simulink model "ex3_k_ss_regulator_sim"  (R2023b)
settings: Solver=ode45  StartTime=0.0  StopTime=t_fin  MaxStep=0.01  RelTol=1e-3
values from neighbouring files (symbols this model uses):
  k = [-20.4 -145.89 -335.994]    [basic_variables.mat]    (also in ex3.m = acker(A, B, sb_vec(i)*ones(1, 3)); ex5.m = acker(A, B, [sb sb sb]); ex6.m = acker(A, B, [sb sb sb]); ex7.m = acker(A, B, [sb sb sb]))
  x_0 = [5 -1 3]    [ex3.m]    (also in ex5.m; ex6.m; ex7.m; extra_ex.m)
settings Model: Creator=vistek528  LastModifiedBy=vistek528
settings DataIOCC: ReturnWorkspaceOutputs=off

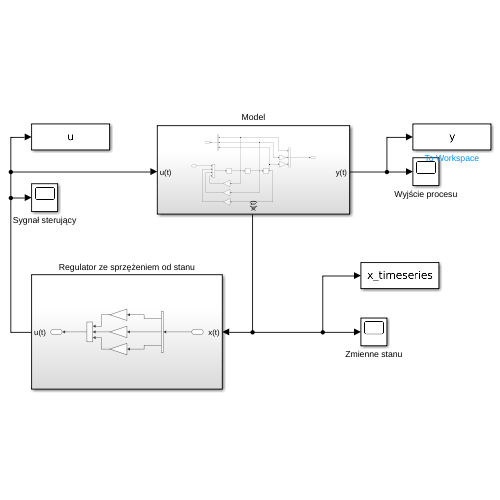
[thumbnail: Simulink's stored preview of the top-level diagram]
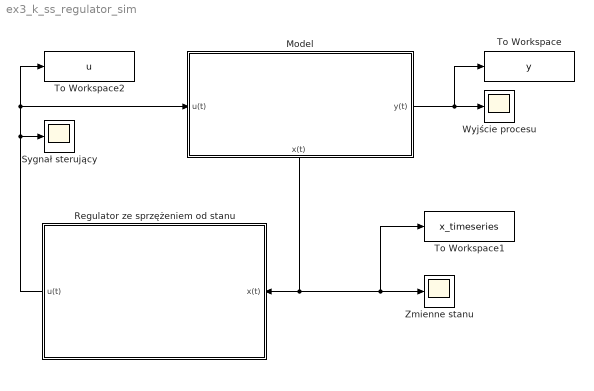
== system ex3_k_ss_regulator_sim ==
  Model : Subsystem
      settings: PortSchema="{\"entries\":[{\"content\":{\"sides\":[{\"content\":{\"connectorIds\":[\"In1\"]},\"type\":\"ConnectorPlacement.EquallySpacedRectSide\",\"uuid\":\"005622f6-1dbe-4fa8-b059-9458e8899b96\"},{\"content\":{\"connectorIds\":[\"Out1\"],\"side\":\"RIGHT\"},\"type\":\"ConnectorPlacement.EquallySpacedRectSide\",\"uuid\":\"7350b0ed-336f-40bc-b296-6ad5a9a87142\"},{\"content\":{\"side\":\"TOP\"},\"type\":\"ConnectorPlacement.EquallySpacedRectSide\",\"uuid\":\"469de851-2f1c-4e76-a936-9009cf2a41ee\"},{\"content\":{\"connectorIds\":[\"Out2\"],\"side\":\"BOTTOM\"},\"type\":\"ConnectorPlacement.EquallySpacedRectSide\",\"uuid\":\"4504609d-b833-4322-8b26-83c28699072e\"}]},\"type\":\"ConnectorPlacement.EquallySpacedConnector\",\"uuid\":\"c3062eda-feb5-4b9f-bf6b-0b995ea2a385\"}],\"packageUris\":[\"http://schema.mathworks.com/mf0/Connector/R2020b\"],\"version\":\"1.0\"}"
  Regulator ze sprzężeniem od stanu : Subsystem
  Sygnał sterujący : Scope
  To Workspace : ToWorkspace  VariableName=y  SaveFormat=Timeseries  SampleTime=-1
  To Workspace1 : ToWorkspace  VariableName=x_timeseries  SaveFormat=Timeseries  SampleTime=-1
  To Workspace2 : ToWorkspace  VariableName=u  SaveFormat=Timeseries  SampleTime=-1
  Wyjście procesu : Scope
  Zmienne stanu : Scope
  wires:
  Regulator ze sprzężeniem od stanu/1(u(t)) -> To Workspace2/1, Model/1(u(t)), Sygnał sterujący/1
  Model/2(x(t)) -> To Workspace1/1, Zmienne stanu/1, Regulator ze sprzężeniem od stanu/1(x(t))
  Model/1(y(t)) -> To Workspace/1, Wyjście procesu/1

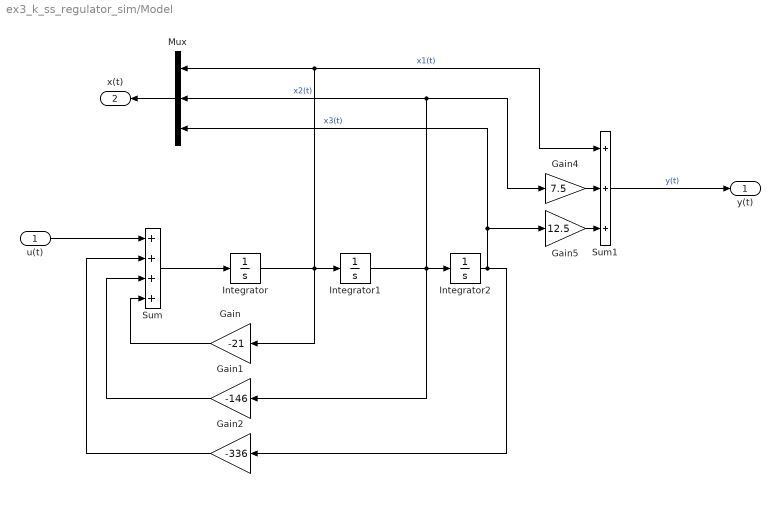
== system ex3_k_ss_regulator_sim/Model ==
  u(t) : Inport
  Gain : Gain  Gain=-21
  Gain1 : Gain  Gain=-146
  Gain2 : Gain  Gain=-336
  Gain4 : Gain  Gain=7.5
  Gain5 : Gain  Gain=12.5
  Integrator : Integrator  InitialCondition=x_0(1)
  Integrator1 : Integrator  InitialCondition=x_0(2)
  Integrator2 : Integrator  InitialCondition=x_0(3)
  Mux : Mux  Inputs=3
  Sum : Sum  Inputs=++++
  Sum1 : Sum  Inputs=+++
  y(t) : Outport
  x(t) : Outport  Port=2
  wires:
  Gain5/1 -> Sum1/3
  Gain1/1 -> Sum/3
  Gain2/1 -> Sum/2
  Sum/1 -> Integrator/1
  u(t)/1 -> Sum/1
  Gain4/1 -> Sum1/2
  Sum1/1 -> y(t)/1  "y(t)"
  Gain/1 -> Sum/4
  Integrator/1 -> Gain/1, Mux/1, Sum1/1, Integrator1/1  "x1(t)"
  Integrator2/1 -> Mux/3, Gain5/1, Gain2/1  "x3(t)"
  Integrator1/1 -> Mux/2, Gain4/1, Gain1/1, Integrator2/1  "x2(t)"
  Mux/1 -> x(t)/1

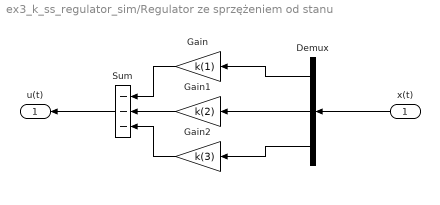
== system ex3_k_ss_regulator_sim/Regulator ze sprzężeniem od stanu ==
  x(t) : Inport
  Demux : Demux  Outputs=3
  Gain : Gain  Gain=k(1)
  Gain1 : Gain  Gain=k(2)
  Gain2 : Gain  Gain=k(3)
  Sum : Sum  Inputs=---
  u(t) : Outport
  wires:
  Demux/3 -> Gain2/1
  Gain/1 -> Sum/1
  Demux/2 -> Gain1/1
  Gain1/1 -> Sum/2
  x(t)/1 -> Demux/1
  Demux/1 -> Gain/1
  Gain2/1 -> Sum/3
  Sum/1 -> u(t)/1
